simulink model "ssc_car_FuelCell1Motor"  (R2020b)
settings: Solver=daessc  StartTime=0.0  StopTime=195  FixedStep=1e-3  RelTol=1e-3  AbsTol=1e-3
InitFcn:
  | Vehicle = sm_car_vehcfg_checkConfig(Vehicle);
undefined symbols (not defined in the file or in its folder): Init
libraries: sdl_lib x10, nesl_utility x9, fl_lib x8, sm_lib x2, Driver_Drive_Cycle x1, Control_FuelCell1Motor x1, Power_FuelCell1Motor x1
Description:
  | Vehicle with Fuel Cell Powertrain
  | 
  | Copyright 2020 The MathWorks, Inc.
settings Model: PauseTimes=10  OrderedModelArguments=off  Creator=jrodgers  LastModifiedBy=smiller
settings SolverCC: AutoScaleAbsTol=off  MaxConsecutiveMinStep=5  SolverJacobianMethodControl=SparsePerturbation
settings DataIOCC: SaveFormat=StructureWithTime  ReturnWorkspaceOutputs=off  SignalLoggingName=logsout_ssc_FuelCell1Motor  ReturnWorkspaceOutputsName=dataOut
settings DebuggingCC: IgnoredZcDiagnostic=none  ArithmeticOperatorsInVariantConditions=warning
settings SFSimCC: CustomCodeUndefinedFunction=UseInterfaceOnly
settings SimscapeCC: SimscapeNominalValues="[{\"value\":\"1\",\"unit\":\"A\"},{\"value\":\"1\",\"unit\":\"bar\"},{\"value\":\"1\",\"unit\":\"cm^2\"},{\"value\":\"1\",\"unit\":\"cm^3/s\"},{\"value\":\"5e6\",\"unit\":\"J/kg\"},{\"value\":\"1\",\"unit\":\"kW\"},{\"value\":\"1\",\"unit\":\"l\"},{\"value\":\"1\",\"unit\":\"N\"},{\"value\":\"1\",\"unit\":\"N*m\"},{\"value\":\"400\",\"unit\":\"V\"},{\"value\":\"355\",\"unit\":\"K\"}]"  SimscapeLogType=all  SimscapeLogSimulationStatistics=on  SimscapeLogName=simlog_ssc_FuelCell1Motor  SimscapeLogLimitData=off
settings ExplorerConfigSet: SimMechanicsOpenEditorOnUpdate=off

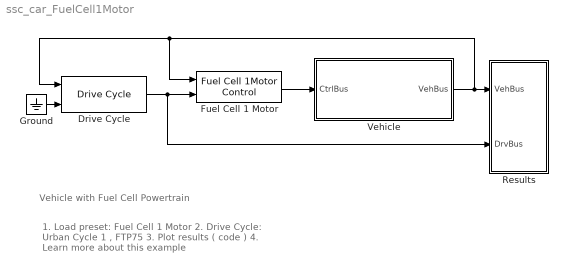
== system ssc_car_FuelCell1Motor ==
  note: 1. Load preset: Fuel Cell 1 Motor
      | 2. Drive Cycle: Urban Cycle 1 , FTP75
      | 3. Plot results ( code )
      | 4. Learn more about this example
  note: Vehicle with Fuel Cell Powertrain
  Drive Cycle : Driver_Drive_Cycle/Drive Cycle  SystemSampleTime=-1  VariantControl=Drive_Cycle  VariantActivationTime=update diagram  Latency=0  AutoFrameSizeCalculation=off
  Fuel Cell 1 Motor : Control_FuelCell1Motor/Fuel Cell 1Motor Control  VariantControl=FuelCell1Motor  Control=Control.FuelCell1Motor
  Ground : Ground
  Results : Subsystem
  Vehicle : Subsystem  mask{Vehicle=Vehicle}
      mask prompts: Vehicle "Vehicle (Structure)"
      mask Display: image('ssc_vehicle_fuel_cell_1motor_vehicle_IMAGE.png');
  wires:
  Vehicle/1(VehBus) -> Drive Cycle/1, Fuel Cell 1 Motor/1, Results/1(VehBus)
  Fuel Cell 1 Motor/1 -> Vehicle/1(CtrlBus)
  Ground/1 -> Drive Cycle/2
  Drive Cycle/1 -> Results/2(DrvBus), Fuel Cell 1 Motor/2

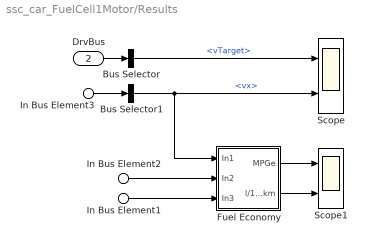
== system ssc_car_FuelCell1Motor/Results ==
  In Bus Element3 : Inport  PortName=VehBus
  In Bus Element2 : Inport  PortName=VehBus  Element=Power.FuelCell.i
  In Bus Element1 : Inport  PortName=VehBus  Element=Power.Battery.Power
  DrvBus : Inport  Port=2
  Bus Selector : BusSelector  OutputSignals=Reference.vTarget
  Bus Selector1 : BusSelector  OutputSignals=Chassis.Body.CG.vx
  Fuel Economy : Subsystem
  Scope : Scope  NumInputPorts=2
  Scope1 : Scope  NumInputPorts=2
  wires:
  DrvBus/1 -> Bus Selector/1
  Bus Selector/1 -> Scope/1  "<vTarget>"
  In Bus Element3/1 -> Bus Selector1/1
  Bus Selector1/1 -> Fuel Economy/1(In1), Scope/2  "<vx>"
  In Bus Element2/1 -> Fuel Economy/2(In2)
  In Bus Element1/1 -> Fuel Economy/3(In3)
  Fuel Economy/1(MPGe) -> Scope1/1
  Fuel Economy/2(l/100km) -> Scope1/2

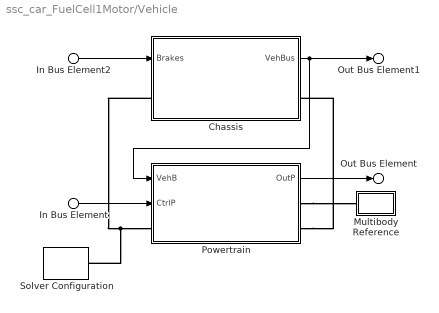
== system ssc_car_FuelCell1Motor/Vehicle ==
  In Bus Element : Inport  PortName=CtrlBus  Element=Power
  In Bus Element2 : Inport  PortName=CtrlBus  Element=Brakes
  Chassis : Subsystem  VariantControl=Full
      mask Display: image('ssc_vehicle_fuel_cell_1motor_chassis_IMAGE.png');
  Multibody Reference : Subsystem
  Powertrain : Subsystem  mask{Powertrain=Vehicle.Powertrain}
      mask prompts: Powertrain "Powertrain (structure)"
      mask Display: image('ssc_vehicle_fuel_cell_1motor_powertrain_IMAGE.png');
  Solver Configuration : nesl_utility/Solver Configuration  PhysicalDomain=network_engine_domain  SubClassName=solver  LeftPortType=input  RightPortType=generic  Tones=[]  Harmonics=[]  SimulateNoise=off  Profile=off  UseLocalSampling=off  EnableSwitchedLinearOptims=on  FrequencyDomain=off  UseCCode=off  RelTol=0.001  AbsTol=1e-06  MinStep=1e-09  ToWorkspace=off  RevertToSquareIcSolve=off  NumHomotopyIterations=100  PhasorMode=off  PhasorModeNumHarmonics=1  DoDC=off  ResidualTolerance=1e-09  UseLocalSolver=off  LocalSolverChoice=NE_BACKWARD_EULER_ADVANCER  LocalSolverSampleTime=0.001  DoFixedCost=off  MaxNonlinIter=3  MaxModeIter=2  LinearAlgebra=auto  EquationFormulation=NE_TIME_EF  DelaysMemoryBudget=1024  AutomaticFiltering=on  FilteringTimeConstant=0.001  PartitionStorageMethod=AS_NEEDED  PartitionMemoryBudget=1024
  Out Bus Element : Outport  PortName=VehBus  Element=Power
  Out Bus Element1 : Outport  PortName=VehBus  Element=Chassis
  wires:
  Powertrain/1(OutP) -> Out Bus Element/1
  In Bus Element2/1 -> Chassis/1(Brakes)
  In Bus Element/1 -> Powertrain/2(CtrlP)
  Chassis/1(VehBus) -> Out Bus Element1/1, Powertrain/1(VehB)
  connections:
  Powertrain/RConn2 -- Chassis/RConn1
  Powertrain/RConn1 -- Multibody Reference/RConn1
  Chassis/LConn1 -- Solver Configuration/RConn1 -- Powertrain/LConn1

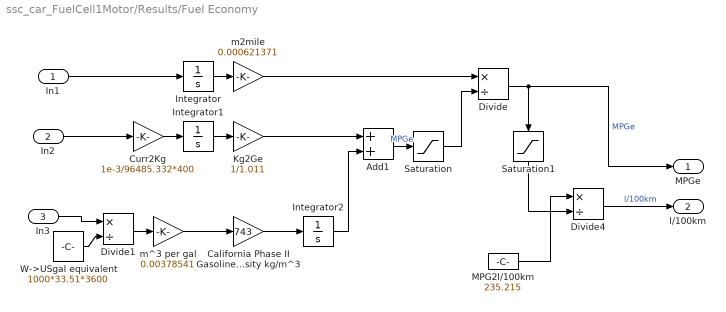
== system ssc_car_FuelCell1Motor/Results/Fuel Economy ==
  In1 : Inport
  In2 : Inport  Port=2
  In3 : Inport  Port=3
  Add1 : Sum
  California Phase II Gasoline density kg/m^3 : Gain  Gain=743
  Curr2Kg : Gain  Gain=1e-3/96485.332*400
  Divide : Product  Inputs=*/
  Divide1 : Product  Inputs=*/
  Divide4 : Product  Inputs=*/
  Integrator : Integrator
  Integrator1 : Integrator
  Integrator2 : Integrator
  Kg2Ge : Gain  Gain=1/1.011
  MPG2l/100km : Constant  Value=235.215
  Saturation : Saturate  UpperLimit=inf  LowerLimit=0.0001
  Saturation1 : Saturate  UpperLimit=inf  LowerLimit=10
  W->USgal equivalent : Constant  Value=1000*33.51*3600
  m2mile : Gain  Gain=0.000621371
  m^3 per gal : Gain  Gain=0.00378541
  MPGe : Outport  VectorParamsAs1DForOutWhenUnconnected=off
  l/100km : Outport  Port=2  VectorParamsAs1DForOutWhenUnconnected=off
  wires:
  MPG2l/100km/1 -> Divide4/1
  m^3 per gal/1 -> California Phase II Gasoline density kg/m^3/1
  Divide4/1 -> l/100km/1  "l/100km"
  Integrator/1 -> m2mile/1
  Divide/1 -> MPGe/1, Saturation1/1  "MPGe"
  Saturation/1 -> Divide/2
  In2/1 -> Curr2Kg/1
  California Phase II Gasoline density kg/m^3/1 -> Integrator2/1
  Add1/1 -> Saturation/1  "MPGe"
  In1/1 -> Integrator/1
  Integrator2/1 -> Add1/2
  W->USgal equivalent/1 -> Divide1/2
  m2mile/1 -> Divide/1
  Saturation1/1 -> Divide4/2
  Curr2Kg/1 -> Integrator1/1
  Kg2Ge/1 -> Add1/1
  Divide1/1 -> m^3 per gal/1
  Integrator1/1 -> Kg2Ge/1
  In3/1 -> Divide1/1

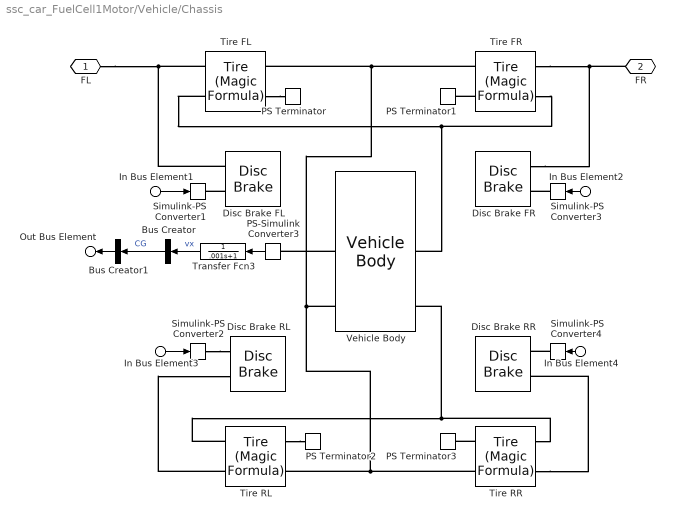
== system ssc_car_FuelCell1Motor/Vehicle/Chassis ==
  In Bus Element1 : Inport  PortName=Brakes  Element=pBrakeFL
  In Bus Element2 : Inport  PortName=Brakes  Element=pBrakeFR
  In Bus Element3 : Inport  PortName=Brakes  Element=pBrakeRL
  In Bus Element4 : Inport  PortName=Brakes  Element=pBrakeRR
  Bus Creator : BusCreator  Inputs=1
  Bus Creator1 : BusCreator  Inputs=1
  Disc Brake FL : sdl_lib/Brakes & Detents/Rotational/Disc Brake  r_mean=Vehicle.Brakes.Front.DiscAndPad.lMeanRadius.Value m  bore=Vehicle.Brakes.Front.Caliper.lCylinderDiameter.Value m  n_pads=Vehicle.Brakes.Front.DiscAndPad.NPads.Value  mu_static=Vehicle.Brakes.Front.DiscAndPad.rMuStatic.Value  mu_coulomb=Vehicle.Brakes.Front.DiscAndPad.rMuKinetic.Value  brkwy_vel=0.1 rad/s  visc_coef=0.001 N*m/(rad/s)  temperature_TLU=[280, 300, 320] K  mu_static_TLU=[.9, .8, .7]  mu_coulomb_TLU=[.8, .7, .6]  thermal_mass=50 kJ/K  temperature_specify=off  temperature_priority=High  temperature=300 K  temperature_nominal_specify=off  temperature_nominal_unit=K  temperature_nominal_value=1
      settings: SourceProductBaseCode=LD
  Disc Brake FR : sdl_lib/Brakes & Detents/Rotational/Disc Brake  r_mean=Vehicle.Brakes.Front.DiscAndPad.lMeanRadius.Value m  bore=Vehicle.Brakes.Front.Caliper.lCylinderDiameter.Value m  n_pads=Vehicle.Brakes.Front.DiscAndPad.NPads.Value  mu_static=Vehicle.Brakes.Front.DiscAndPad.rMuStatic.Value  mu_coulomb=Vehicle.Brakes.Front.DiscAndPad.rMuKinetic.Value  brkwy_vel=0.1 rad/s  visc_coef=0.001 N*m/(rad/s)  temperature_TLU=[280, 300, 320] K  mu_static_TLU=[.9, .8, .7]  mu_coulomb_TLU=[.8, .7, .6]  thermal_mass=50 kJ/K  temperature_specify=off  temperature_priority=High  temperature=300 K  temperature_nominal_specify=off  temperature_nominal_unit=K  temperature_nominal_value=1
      settings: SourceProductBaseCode=LD
  Disc Brake RL : sdl_lib/Brakes & Detents/Rotational/Disc Brake  r_mean=Vehicle.Brakes.Front.DiscAndPad.lMeanRadius.Value m  bore=Vehicle.Brakes.Front.Caliper.lCylinderDiameter.Value m  n_pads=Vehicle.Brakes.Front.DiscAndPad.NPads.Value  mu_static=Vehicle.Brakes.Front.DiscAndPad.rMuStatic.Value  mu_coulomb=Vehicle.Brakes.Front.DiscAndPad.rMuKinetic.Value  brkwy_vel=0.1 rad/s  visc_coef=0.001 N*m/(rad/s)  temperature_TLU=[280, 300, 320] K  mu_static_TLU=[.9, .8, .7]  mu_coulomb_TLU=[.8, .7, .6]  thermal_mass=50 kJ/K  temperature_specify=off  temperature_priority=High  temperature=300 K  temperature_nominal_specify=off  temperature_nominal_unit=K  temperature_nominal_value=1
      settings: SourceProductBaseCode=LD
  Disc Brake RR : sdl_lib/Brakes & Detents/Rotational/Disc Brake  r_mean=Vehicle.Brakes.Front.DiscAndPad.lMeanRadius.Value m  bore=Vehicle.Brakes.Front.Caliper.lCylinderDiameter.Value m  n_pads=Vehicle.Brakes.Front.DiscAndPad.NPads.Value  mu_static=Vehicle.Brakes.Front.DiscAndPad.rMuStatic.Value  mu_coulomb=Vehicle.Brakes.Front.DiscAndPad.rMuKinetic.Value  brkwy_vel=0.1 rad/s  visc_coef=0.001 N*m/(rad/s)  temperature_TLU=[280, 300, 320] K  mu_static_TLU=[.9, .8, .7]  mu_coulomb_TLU=[.8, .7, .6]  thermal_mass=50 kJ/K  temperature_specify=off  temperature_priority=High  temperature=300 K  temperature_nominal_specify=off  temperature_nominal_unit=K  temperature_nominal_value=1
      settings: SourceProductBaseCode=LD
  PS Terminator{,1..3} (4 alike) : fl_lib/Physical Signals/Sinks/PS Terminator
  PS-Simulink Converter3 : nesl_utility/PS-Simulink Converter  PhysicalDomain=network_engine_domain  SubClassName=ps_output  LeftPortType=input  RightPortType=output  PseudoPeriodic=off  Frequencies=[]  Unit=m/s  AffineConversion=off
  Simulink-PS Converter{1..4} (4 alike) : nesl_utility/Simulink-PS Converter  PhysicalDomain=network_engine_domain  SubClassName=ps_input  LeftPortType=input  RightPortType=output  PseudoPeriodic=off  Frequencies=[]  NoiseDistribution=none  NoiseParameters=[]  Unit=bar  AffineConversion=off  FilteringAndDerivatives=provide  SimscapeFilterOrder=1  InputFilterTimeConstant=0.01  UdotUserProvided=0
  Tire FL : sdl_lib/Tires & Vehicles/Tire (Magic Formula)  parameterization=1  F_z1=3000 N  F_x1=3500 N  kappa1=6  B_m=10  C_m=1.9  D_m=1  E_m=0.97  fz0=4e+3 N  p_Cx=1.685  p_Dx=[ 1.21 -0.037 ]  p_Ex=[ 0.344 0.095 -0.02 0 ]  p_Kx=[ 21.51 -0.163 0.245 ]  p_Hx=[ -0.002 0.002 ]  p_Vx=[ 0 0 ]  v_tr_thr=0.1 m/s  r_e=Vehicle.Chassis.TireF.tire_radius.Value m  model_compliance=0  stiffness=1e+6 N/m  damping=1000 N/(m/s)  model_inertia=1  inertia=Vehicle.Chassis.TireF.Inertia.Value(1) kg*m^2  initial_velocity=Init.Front.nWheel.Value(1) rad/s  model_resistance=1  resistance_model=1  coeff=0.015  p_tire=250e3 Pa  alpha=-0.003  beta=0.97  coeff_a=84e-4  coeff_b=6.2e-4 s/m  coeff_c=1.6e-4 s^2/m^2  v_thr=1e-3 m/s
  Tire FR : sdl_lib/Tires & Vehicles/Tire (Magic Formula)  parameterization=1  F_z1=3000 N  F_x1=3500 N  kappa1=6  B_m=10  C_m=1.9  D_m=1  E_m=0.97  fz0=4e+3 N  p_Cx=1.685  p_Dx=[ 1.21 -0.037 ]  p_Ex=[ 0.344 0.095 -0.02 0 ]  p_Kx=[ 21.51 -0.163 0.245 ]  p_Hx=[ -0.002 0.002 ]  p_Vx=[ 0 0 ]  v_tr_thr=0.1 m/s  r_e=Vehicle.Chassis.TireF.tire_radius.Value m  model_compliance=0  stiffness=1e+6 N/m  damping=1000 N/(m/s)  model_inertia=1  inertia=Vehicle.Chassis.TireF.Inertia.Value(1) kg*m^2  initial_velocity=Init.Front.nWheel.Value(1) rad/s  model_resistance=1  resistance_model=1  coeff=0.015  p_tire=250e3 Pa  alpha=-0.003  beta=0.97  coeff_a=84e-4  coeff_b=6.2e-4 s/m  coeff_c=1.6e-4 s^2/m^2  v_thr=1e-3 m/s
  Tire RL : sdl_lib/Tires & Vehicles/Tire (Magic Formula)  parameterization=1  F_z1=3000 N  F_x1=3500 N  kappa1=6  B_m=10  C_m=1.9  D_m=1  E_m=0.97  fz0=4e+3 N  p_Cx=1.685  p_Dx=[ 1.21 -0.037 ]  p_Ex=[ 0.344 0.095 -0.02 0 ]  p_Kx=[ 21.51 -0.163 0.245 ]  p_Hx=[ -0.002 0.002 ]  p_Vx=[ 0 0 ]  v_tr_thr=0.1 m/s  r_e=Vehicle.Chassis.TireF.tire_radius.Value m  model_compliance=0  stiffness=1e+6 N/m  damping=1000 N/(m/s)  model_inertia=1  inertia=Vehicle.Chassis.TireF.Inertia.Value(1) kg*m^2  initial_velocity=Init.Front.nWheel.Value(1) rad/s  model_resistance=1  resistance_model=1  coeff=0.015  p_tire=250e3 Pa  alpha=-0.003  beta=0.97  coeff_a=84e-4  coeff_b=6.2e-4 s/m  coeff_c=1.6e-4 s^2/m^2  v_thr=1e-3 m/s
  Tire RR : sdl_lib/Tires & Vehicles/Tire (Magic Formula)  parameterization=1  F_z1=3000 N  F_x1=3500 N  kappa1=6  B_m=10  C_m=1.9  D_m=1  E_m=0.97  fz0=4e+3 N  p_Cx=1.685  p_Dx=[ 1.21 -0.037 ]  p_Ex=[ 0.344 0.095 -0.02 0 ]  p_Kx=[ 21.51 -0.163 0.245 ]  p_Hx=[ -0.002 0.002 ]  p_Vx=[ 0 0 ]  v_tr_thr=0.1 m/s  r_e=Vehicle.Chassis.TireF.tire_radius.Value m  model_compliance=0  stiffness=1e+6 N/m  damping=1000 N/(m/s)  model_inertia=1  inertia=Vehicle.Chassis.TireF.Inertia.Value(1) kg*m^2  initial_velocity=Init.Front.nWheel.Value(1) rad/s  model_resistance=1  resistance_model=1  coeff=0.015  p_tire=250e3 Pa  alpha=-0.003  beta=0.97  coeff_a=84e-4  coeff_b=6.2e-4 s/m  coeff_c=1.6e-4 s^2/m^2  v_thr=1e-3 m/s
  Transfer Fcn3 : TransferFcn  Denominator=[.001 1]
  Vehicle Body : sdl_lib/Tires & Vehicles/Vehicle Body  mass=Vehicle.Chassis.Body.m.Value kg  n_w=2  x_f=Vehicle.Chassis.Body.sAxleF.Value(1)-Vehicle.Chassis.Body.sCG.Value(1) m  x_r=-Vehicle.Chassis.Body.sAxleR.Value(1)+Vehicle.Chassis.Body.sCG.Value(1) m  y_c=Vehicle.Chassis.Body.sCG.Value(3)-Vehicle.Chassis.Body.sAxleF.Value(3) m  model_pitch=0  inertia=4000 kg*m^2  suspension_model=1  k_f=1e4 N/m  b_f=1e4 N/(m/s)  k_r=1e4 N/m  b_r=1e4 N/(m/s)  k_f_TLU=[-2000, -1000, 0, 1000, 2000] N  x_f_TLU=[-.4, -.2, 0, .2, .4] m  b_f_TLU=[-200, -100, 0, 100, 200] N  v_f_TLU=[-4, -2, 0, 2, 4] m/s  k_r_TLU=[-2000, -1000, 0, 1000, 2000] N  x_r_TLU=[-.4, -.2, 0, .2, .4] m  b_r_TLU=[-200, -100, 0, 100, 200] N  v_r_TLU=[-4, -2, 0, 2, 4] m/s  interp_method=simscape.enum.interpolation.linear  extrap_method=simscape.enum.extrapolation.linear  model_hardstop=0  upper_bound_f=.25 m  lower_bound_f=-.25 m  stop_k_f=1e6 N/m  stop_b_f=150 N/(m/s)  upper_bound_r=.25 m  lower_bound_r=-.25 m  stop_k_r=1e6 N/m  stop_b_r=150 N/(m/s)  initial_pitch=0 rad  initial_pitch_rate=0 rad/s  g=9.81 m/s^2  liftoff_warning=0  area=Vehicle.Chassis.Aero.ARef.Value m^2  Cd=Vehicle.Chassis.Aero.CD.Value  rho=1.18 kg/m^3  v_specify=on  v_priority=High  v=Init.Chassis.vChassis.Value(1) m/s  v_nominal_specify=off  v_nominal_unit=m/s  v_nominal_value=1
  FL : PMIOPort  Side=Left
  FR : PMIOPort  Port=2  Side=Right
  Out Bus Element : Outport  PortName=VehBus  Element=Body
  wires:
  PS-Simulink Converter3/1 -> Transfer Fcn3/1
  Transfer Fcn3/1 -> Bus Creator/1  "vx"
  In Bus Element1/1 -> Simulink-PS Converter1/1
  Bus Creator/1 -> Bus Creator1/1  "CG"
  Bus Creator1/1 -> Out Bus Element/1
  In Bus Element3/1 -> Simulink-PS Converter2/1
  In Bus Element2/1 -> Simulink-PS Converter3/1
  In Bus Element4/1 -> Simulink-PS Converter4/1
  connections:
  Disc Brake FL/LConn1 -- Simulink-PS Converter1/RConn1
  Tire FL/LConn2 -- FL/RConn1 -- Disc Brake FL/LConn2
  Tire FL/RConn1 -- PS Terminator/LConn1
  Vehicle Body/LConn2 -- PS-Simulink Converter3/LConn1
  Tire FL/LConn1 -- Tire FR/LConn1 -- Vehicle Body/RConn2
  Tire RR/RConn2 -- Tire RL/RConn2 -- Vehicle Body/LConn1 -- Tire FR/RConn2 -- Tire FL/RConn2
  Disc Brake FR/LConn2 -- Tire FR/LConn2 -- FR/RConn1
  Tire FR/RConn1 -- PS Terminator1/LConn1
  Tire RL/LConn2 -- Disc Brake RL/LConn2
  Tire RR/LConn1 -- Tire RL/LConn1 -- Vehicle Body/RConn1
  Tire RR/LConn2 -- Disc Brake RR/LConn2
  Tire RL/RConn1 -- PS Terminator2/LConn1
  Tire RR/RConn1 -- PS Terminator3/LConn1
  Simulink-PS Converter2/RConn1 -- Disc Brake RL/LConn1
  Simulink-PS Converter3/RConn1 -- Disc Brake FR/LConn1
  Simulink-PS Converter4/RConn1 -- Disc Brake RR/LConn1

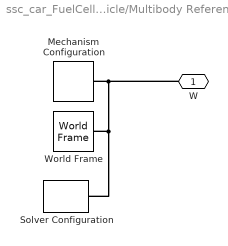
== system ssc_car_FuelCell1Motor/Vehicle/Multibody Reference ==
  Mechanism Configuration : sm_lib/Utilities/Mechanism Configuration  UniformGravity=Constant  GravityVector=[0 0 -9.80665]  GravityUnits=m/s^2  LinearizationDelta=0.001
  Solver Configuration : nesl_utility/Solver Configuration  PhysicalDomain=network_engine_domain  SubClassName=solver  LeftPortType=input  RightPortType=generic  Tones=[]  Harmonics=[]  SimulateNoise=off  Profile=off  UseLocalSampling=off  EnableSwitchedLinearOptims=on  FrequencyDomain=off  UseCCode=off  RelTol=0.001  AbsTol=1e-06  MinStep=1e-09  ToWorkspace=off  RevertToSquareIcSolve=off  NumHomotopyIterations=100  PhasorMode=off  PhasorModeNumHarmonics=1  DoDC=off  ResidualTolerance=1e-09  UseLocalSolver=off  LocalSolverChoice=NE_BACKWARD_EULER_ADVANCER  LocalSolverSampleTime=0.001  DoFixedCost=off  MaxNonlinIter=3  MaxModeIter=2  LinearAlgebra=auto  EquationFormulation=NE_TIME_EF  DelaysMemoryBudget=1024  AutomaticFiltering=on  FilteringTimeConstant=0.001  PartitionStorageMethod=AS_NEEDED  PartitionMemoryBudget=1024
  World Frame : sm_lib/Frames and Transforms/World Frame
  W : PMIOPort  Side=Right
  connections:
  Mechanism Configuration/RConn1 -- W/RConn1 -- Solver Configuration/RConn1 -- World Frame/RConn1

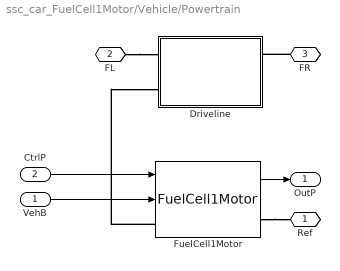
== system ssc_car_FuelCell1Motor/Vehicle/Powertrain ==
  VehB : Inport
  CtrlP : Inport  Port=2
  Driveline : Subsystem
      mask Display: image('ssc_vehicle_fuel_cell_1motor_driveline_IMAGE.png');
  FuelCell1Motor : Power_FuelCell1Motor/FuelCell1Motor  VariantControl=FuelCell1Motor  Power=Powertrain.Power
  Ref : PMIOPort  Side=Right
  FL : PMIOPort  Port=2  Side=Left
  FR : PMIOPort  Port=3  Side=Right
  OutP : Outport  VectorParamsAs1DForOutWhenUnconnected=off
  wires:
  FuelCell1Motor/1 -> OutP/1
  CtrlP/1 -> FuelCell1Motor/1
  VehB/1 -> FuelCell1Motor/2
  connections:
  FuelCell1Motor/LConn1 -- Driveline/LConn2
  FuelCell1Motor/RConn1 -- Ref/RConn1
  FL/RConn1 -- Driveline/LConn1
  FR/RConn1 -- Driveline/RConn1

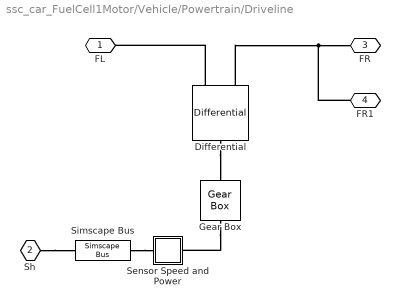
== system ssc_car_FuelCell1Motor/Vehicle/Powertrain/Driveline ==
  Differential : sdl_lib/Gears/Differential  driveshaft_location=2  cd_ratio=Vehicle.Powertrain.Driveline.DifferentialF.ratio.Value  friction_model=1  efficiency=[.85, .92]  mu_visc=[0, 0] N*m/(rad/s)  pwr_thr=[.001, .001] W  carrier_inertia=0 kg*m^2  planet_inertia=0 kg*m^2  temperature_TLU=[280, 300, 320] K  efficiency_ss_TLU=[.95, .9, .85]  efficiency_cd_TLU=[.95, .9, .85]  thermal_mass=50 J/K  T_init=300 K
      settings: SourceProductBaseCode=LD
  Gear Box : fl_lib/Mechanical/Mechanisms/Gear Box  ratio=Vehicle.Powertrain.Driveline.GearboxF.ratio.Value  t_in_specify=off  t_in_priority=None  t_in=0 N*m  t_in_nominal_specify=off  t_in_nominal_unit=N*m  t_in_nominal_value=1  t_out_specify=off  t_out_priority=None  t_out=0 N*m  t_out_nominal_specify=off  t_out_nominal_unit=N*m  t_out_nominal_value=1
  Sensor Speed and Power : Subsystem
      mask Display: disp('S')
  Simscape Bus : SimscapeBus  HierarchyStrings=ShaftF
  FL : PMIOPort  Side=Left
  Sh : PMIOPort  Port=2  Side=Left
  FR : PMIOPort  Port=3  Side=Right
  FR1 : PMIOPort  Port=4  Side=Right
  connections:
  Gear Box/LConn1 -- Sensor Speed and Power/RConn1
  Simscape Bus/LConn1 -- Sensor Speed and Power/LConn1
  Differential/RConn2 -- FL/RConn1
  Sh/RConn1 -- Simscape Bus/RConn1
  Differential/RConn1 -- FR1/RConn1 -- FR/RConn1
  Differential/LConn1 -- Gear Box/RConn1

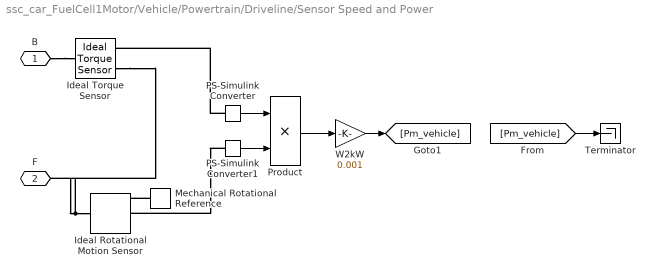
== system ssc_car_FuelCell1Motor/Vehicle/Powertrain/Driveline/Sensor Speed and Power ==
  Ideal Rotational Motion Sensor : fl_lib/Mechanical/Mechanical Sensors/Ideal Rotational Motion Sensor  offset=0 rad
  Ideal Torque Sensor : fl_lib/Mechanical/Mechanical Sensors/Ideal Torque Sensor
  Mechanical Rotational Reference : fl_lib/Mechanical/Rotational Elements/Mechanical Rotational Reference
  PS-Simulink Converter : nesl_utility/PS-Simulink Converter  PhysicalDomain=network_engine_domain  SubClassName=ps_output  LeftPortType=input  RightPortType=output  PseudoPeriodic=off  Frequencies=[]  Unit=N*m  AffineConversion=off
  PS-Simulink Converter1 : nesl_utility/PS-Simulink Converter  PhysicalDomain=network_engine_domain  SubClassName=ps_output  LeftPortType=input  RightPortType=output  PseudoPeriodic=off  Frequencies=[]  Unit=rad/s  AffineConversion=off
  Product : Product  RndMeth=Zero
  Terminator : Terminator
  W2kW : Gain  Gain=0.001
  B : PMIOPort  Side=Left
  F : PMIOPort  Port=2  Side=Right
  wires:
  W2kW/1 -> [Pm_vehicle]
  Product/1 -> W2kW/1
  PS-Simulink Converter/1 -> Product/1
  PS-Simulink Converter1/1 -> Product/2
  [Pm_vehicle] -> Terminator/1
  connections:
  Mechanical Rotational Reference/LConn1 -- Ideal Rotational Motion Sensor/RConn1
  Ideal Rotational Motion Sensor/LConn1 -- F/RConn1 -- Ideal Torque Sensor/RConn1
  B/RConn1 -- Ideal Torque Sensor/LConn1
  PS-Simulink Converter/LConn1 -- Ideal Torque Sensor/RConn2
  PS-Simulink Converter1/LConn1 -- Ideal Rotational Motion Sensor/RConn2
